simulink model "SEAMOUR_Sim"  (R2023a)
settings: Solver=ode4  StartTime=0.0  StopTime=12  FixedStep=simulation_ts  MaxStep=0.001  MinStep=0.0001  RelTol=1e-3  EnableMultiTasking=on
values from neighbouring files (symbols this model uses):
  Area_y = [0.0031581,0.024875,0.025026,0.021123,0.021123,0.025026,0.024875,0.037486]    [init_file.m]
  Area_z = [0.0031588,0.028932,0.035488,0.030129,0.030129,0.035488,0.028932,0.039984]    [init_file.m]
  Cd_y = [0.5645,0.5232,0.4085,0.3589,0.3589,0.40849,0.5232,0.4642]    [init_file.m]
  Cd_z = [0.5645,0.52,0.5843,0.533,0.533,0.5843,0.52,0.5238]    [init_file.m]
  Coeff = [xudot, yvdot, zwdot]    [init_file.m]
  gravity = 9.81    [init_file.m]
  m = (4*pi*rho*a*b*b)/3    (= 16.3133743522)    [init_file.m]
  offset = 0.002    [init_file.m]
  percent_y = Area_y/t_y    [init_file.m]
  percent_z = Area_z/t_z    [init_file.m]
  xudot = k1*m    [init_file.m]
undefined symbols (not defined in the file or in its folder): center_body, headmain, headmotorshield, headmount, hindconnection, hindcover, kx_lower, kx_upper, kz_lower, kz_upper, lefthindflipper, lefthindmotor, leftmotor1, leftmotor2, leftmotor3, lf_lower, lf_upper, rf_lower, rf_upper, righthindflipper, righthindmotor, rightmotor1, rightmotor2, rightmotor3, tailmotorshield, tailmount, X, Y, Z
libraries: nesl_utility x208, sm_lib x149
(part 1 of 7)
settings Model: Creator=sk3496  LastModifiedBy=andyc
settings SolverCC: InitialStep=0.0001  ExtrapolationOrder=3  AutoInsertRateTranBlk=on  InsertRTBMode=Never (minimum delay)  MinimalZcImpactIntegration=on
settings DataIOCC: LimitDataPoints=on
settings OptimizationCC: LifeSpan=inf
settings DebuggingCC: ReadBeforeWriteMsg=DisableAll  WriteAfterWriteMsg=DisableAll  WriteAfterReadMsg=DisableAll  AlgebraicLoopMsg=none  MultiTaskDSMMsg=none  UnconnectedInputMsg=warning  UnconnectedOutputMsg=warning  UnconnectedLineMsg=warning  AllowSymbolicDim=off  SFUnexpectedBacktrackingDiag=warning  SFNoUnconditionalDefaultTransitionDiag=warning  SFExecutionAtInitializationDiag=none  ArithmeticOperatorsInVariantConditions=warning
settings ModelReferenceCC: UpdateModelReferenceTargets=IfOutOfDate  EnableRefExpFcnMdlSchedulingChecks=on
settings SFSimCC: SFSimEcho=off  SimUseLocalCustomCode=off  CustomCodeUndefinedFunction=UseInterfaceOnly
settings RTWCC: RTWUseLocalCustomCode=off
settings CodeAppCC: StateflowObjectComments=on
settings GRTTargetCC: TargetLangStandard=C89/C90 (ANSI)
settings ConfigComp: CovMetricSettings=dw  CovSaveCumulativeToWorkspaceVar=on  CovSaveSingleToWorkspaceVar=on  CovExternalEMLEnable=off  CovSFcnEnable=off
settings SimscapeCC: SimscapeNominalValues="[{\"value\":\"10\",\"unit\":\"V\"},{\"value\":\"1\",\"unit\":\"A\"},{\"value\":\"10\",\"unit\":\"N*m\"},{\"value\":\"10\",\"unit\":\"bar\"},{\"value\":\"100\",\"unit\":\"kJ/kg\"},{\"value\":\"1\",\"unit\":\"kW\"},{\"value\":\"300\",\"unit\":\"K\"},{\"value\":\"100\",\"unit\":\"cm^3/s\"},{\"value\":\"1\",\"unit\":\"kN\"},{\"value\":\"1\",\"unit\":\"g/cm^3\"},{\"value\":\"1\",\"unit\":\"l\"},{\"value\":\"1\",\"unit\":\"cm^2\"},{\"value\":\"60\",\"unit\":\"Hz\"}]"  SimscapeLogDataHistory=10000
settings ConfigurationSet: Description=SimMechanics 2G

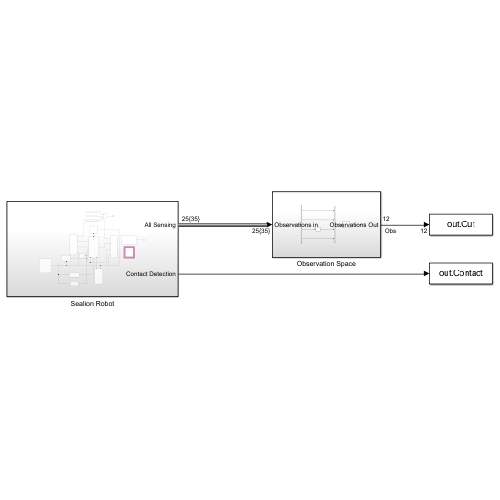
[thumbnail: Simulink's stored preview of the top-level diagram]
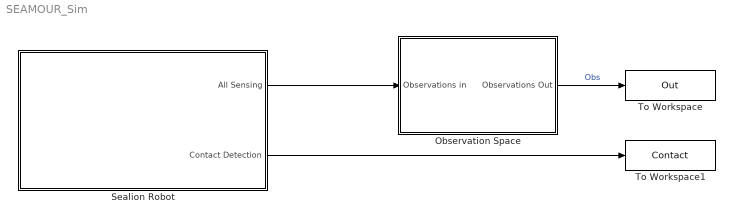
== system SEAMOUR_Sim ==
  Observation Space : Subsystem
  Sealion Robot : Subsystem
  To Workspace : ToWorkspace  VariableName=Out  SaveFormat=Structure  SampleTime=-1
  To Workspace1 : ToWorkspace  VariableName=Contact  SampleTime=-1
      settings: Save2DSignal=2-D array (concatenate along first dimension)
  wires:
  Sealion Robot/1(All Sensing) -> Observation Space/1(Observations in)
  Observation Space/1(Observations Out) -> To Workspace/1  "Obs"
  Sealion Robot/2(Contact Detection) -> To Workspace1/1

== system SEAMOUR_Sim/Observation Space ==
  Observations in : Inport
  Bus Selector : BusSelector  OutputSignals=Body Position/Orientation.Position,Body Position/Orientation.Velocities,Body Position/Orientation.Euler,Body Position/Orientation.AngVel
  Mux : Mux
  Rate Transition : RateTransition
  Reshape1 : Reshape
  Observations Out : Outport
  wires:
  Observations in/1 -> Bus Selector/1
  Bus Selector/3 -> Reshape1/1  "<Euler>"
  Mux/1 -> Rate Transition/1
  Rate Transition/1 -> Observations Out/1
  Bus Selector/1 -> Mux/1  "<Position>"
  Bus Selector/2 -> Mux/2  "<Velocities>"
  Reshape1/1 -> Mux/3
  Bus Selector/4 -> Mux/4  "<AngVel>"

== system SEAMOUR_Sim/Sealion Robot ==
  6 DoF Joint : Subsystem
  All Sesning : Subsystem
  "Allignment Check " : Subsystem
      settings: PortSchema="{\"entries\":[{\"content\":{\"sides\":[{\"content\":{},\"type\":\"ConnectorPlacement.EquallySpacedRectSide\",\"uuid\":\"6b8e2414-6244-4178-ae28-f39780b7a688\"},{\"content\":{\"connectorIds\":[\"RConn1\"],\"side\":\"RIGHT\"},\"type\":\"ConnectorPlacement.EquallySpacedRectSide\",\"uuid\":\"9fd554ac-8ecb-4d79-a032-4bdf23530bdb\"},{\"content\":{\"side\":\"TOP\"},\"type\":\"ConnectorPlacement.EquallySpacedRectSide\",\"uuid\":\"ea6b4beb-e3fc-494d-baa7-bd1cb7ea7a6d\"},{\"content\":{\"connectorIds\":[\"RConn2\"],\"side\":\"BOTTOM\"},\"type\":\"ConnectorPlacement.EquallySpacedRectSide\",\"uuid\":\"7e6024d3-5a2e-46cf-8b0d-4584228e349b\"}]},\"type\":\"ConnectorPlacement.EquallySpacedConnector\",\"uuid\":\"58c9547a-a497-47e7-97e0-14a41819356b\"}],\"packageUris\":[\"http://schema.mathworks.com/mf0/Connector/R2020b\"],\"version\":\"1.0\"}"
  Buoyancy : Subsystem
  Configuration : Subsystem
  Constant : Constant  Value=0
  Distributed Forces : Subsystem
  HEAD : Subsystem
      settings: PortSchema="{\"entries\":[{\"content\":{\"sides\":[{\"content\":{\"connectorIds\":[\"LConn1\"]},\"type\":\"ConnectorPlacement.EquallySpacedRectSide\",\"uuid\":\"8100d47f-b021-448f-a21c-a2dff3a56156\"},{\"content\":{\"side\":\"RIGHT\"},\"type\":\"ConnectorPlacement.EquallySpacedRectSide\",\"uuid\":\"87f545d1-57bd-46af-b957-aab136ed44b5\"},{\"content\":{\"connectorIds\":[\"LConn2\"],\"side\":\"TOP\"},\"type\":\"ConnectorPlacement.EquallySpacedRectSide\",\"uuid\":\"2e5f77fd-6041-45d2-a1f1-1d00d6a46e15\"},{\"content\":{\"side\":\"BOTTOM\"},\"type\":\"ConnectorPlacement.EquallySpacedRectSide\",\"uuid\":\"5c5245d9-55c2-4eb3-8804-cb1ddb21d0c7\"}]},\"type\":\"ConnectorPlacement.EquallySpacedConnector\",\"uuid\":\"e46f37ca-c74f-4ae2-877d-e1d0fe3e0b33\"}],\"packageUris\":[\"http://schema.mathworks.com/mf0/Connector/R2020b\"],\"version\":\"1.0\"}"
      mask Display: image('Icons\Head.PNG')
  LEFT FLIPPER : Subsystem
      settings: PortSchema="{\"entries\":[{\"content\":{\"sides\":[{\"content\":{},\"type\":\"ConnectorPlacement.EquallySpacedRectSide\",\"uuid\":\"08e76363-06a3-4a20-82bd-2cf2d6ca0025\"},{\"content\":{\"side\":\"RIGHT\"},\"type\":\"ConnectorPlacement.EquallySpacedRectSide\",\"uuid\":\"c2e121f7-1b05-4496-8847-526d88e6935b\"},{\"content\":{\"side\":\"TOP\"},\"type\":\"ConnectorPlacement.EquallySpacedRectSide\",\"uuid\":\"ac3d01a4-8d73-45c4-9a34-c3a91121d4c6\"},{\"content\":{\"connectorIds\":[\"RConn1\",\"RConn2\",\"RConn3\",\"RConn4\"],\"side\":\"BOTTOM\"},\"type\":\"ConnectorPlacement.EquallySpacedRectSide\",\"uuid\":\"2a7e8164-9c64-41a5-bf67-24a4b06e045d\"}]},\"type\":\"ConnectorPlacement.EquallySpacedConnector\",\"uuid\":\"d5f6bfd5-69aa-4fea-98cc-f55e388c733b\"}],\"packageUris\":[\"http://schema.mathworks.com/mf0/Connector/R2020b\"],\"version\":\"1.0\"}"
      mask Display: image('Icons\Left_Flipper.PNG')
  PS-Simulink Converter : nesl_utility/PS-Simulink Converter  PhysicalDomain=network_engine_domain  SubClassName=ps_output  LeftPortType=input  RightPortType=output  PseudoPeriodic=off  Frequencies=[]  VectorFormat=inherit  Unit=inherit  AffineConversion=off
  RIGHT FLIPPER : Subsystem
      mask Display: image('Icons\Right_Flipper.PNG')
  Rear : Subsystem
      mask Display: image('Icons\Hind Section.PNG')
  Simulink-PS Converter : nesl_utility/Simulink-PS Converter  PhysicalDomain=network_engine_domain  SubClassName=ps_input  LeftPortType=input  RightPortType=output  PseudoPeriodic=off  Frequencies=[]  NoiseDistribution=none  NoiseParameters=[]  Unit=1  AffineConversion=off  FilteringAndDerivatives=provide  SimscapeFilterOrder=1  InputFilterTimeConstant=0.001  UdotUserProvided=0
  Spatial Contact Force : sm_lib/Forces and Torques/Spatial Contact Force  SenseContactBaseRotation=off  SenseContactBaseTranslation=off  CoefficientOfDynamicFriction=0.3  CoefficientOfStaticFriction=0.5  NormalDamping=1e3  NormalDampingUnits=N/(m/s)  SenseContactSignal=on  NormalStiffness=1e6  NormalStiffnessUnits=N/m  FrictionalCriticalVelocity=1e-3  FrictionalCriticalVelocityUnits=m/s  ZeroCrossDetectContactStartAndEnd=off  SenseContactFollowerRotation=off  SenseContactFollowerTranslation=off  FrictionType=None  SenseFrictionalForceMagnitude=off  SenseNormalForceMagnitude=off  NormalForceType=ProvidedByInput  SenseNormalVelocity=off  SenseSeparationDistance=off  SenseTangentialVelocity=off  NormalTransitionRegionWidth=1e-4  NormalTransitionRegionWidthUnits=m
  Subsystem : Subsystem
      settings: PortSchema="{\"entries\":[{\"content\":{\"sides\":[{\"content\":{\"connectorIds\":[\"LConn1\"]},\"type\":\"ConnectorPlacement.EquallySpacedRectSide\",\"uuid\":\"dcf17234-a2cb-4e8c-ab9b-e151f23c1481\"},{\"content\":{\"connectorIds\":[\"RConn1\",\"RConn2\"],\"side\":\"RIGHT\"},\"type\":\"ConnectorPlacement.EquallySpacedRectSide\",\"uuid\":\"c4f35782-c071-469c-995b-0ee337f7014d\"},{\"content\":{\"connectorIds\":[\"LConn2\"],\"side\":\"TOP\"},\"type\":\"ConnectorPlacement.EquallySpacedRectSide\",\"uuid\":\"5f61ab44-4bc3-42d8-956e-937e7208d291\"},{\"content\":{\"connectorIds\":[\"RConn3\",\"RConn4\",\"RConn5\"],\"side\":\"BOTTOM\"},\"type\":\"ConnectorPlacement.EquallySpacedRectSide\",\"uuid\":\"463c5b41-6d5a-4342-9fda-0edfa9c3fa23\"}]},\"type\":\"ConnectorPlacement.EquallySpacedConnector\",\"uuid\":\"cfa1c9cb-cfd7-41ad-9d03-2a28f55bccb4\"}],\"packageUris\":[\"http://schema.mathworks.com/mf0/Connector/R2020b\"],\"version\":\"1.0\"}"
      mask Display: image('Icons\Center Body.PNG')
  Sum : Sum  Inputs=+++
  Trajectory Inputs : Subsystem
  All Sensing : Outport
  Contact Detection : Outport  Port=2
  wires:
  All Sesning/1(All Sensing) -> All Sensing/1
  Constant/1 -> Simulink-PS Converter/1
  PS-Simulink Converter/1 -> Sum/3
  [Right_Foreflipper_Contact] -> Sum/2
  [Left_Foreflipper_Contact] -> Sum/1
  Sum/1 -> Contact Detection/1
  connections:
  RIGHT FLIPPER/LConn2 -- Subsystem/LConn1
  LEFT FLIPPER/RConn3 -- Subsystem/RConn1
  Buoyancy/LConn1 -- 6 DoF Joint/RConn1 -- "Allignment Check "/RConn1 -- Subsystem/RConn2
  Rear/LConn1 -- Subsystem/RConn3
  HEAD/LConn2 -- Subsystem/LConn2
  Configuration/RConn1 -- HEAD/LConn1 -- RIGHT FLIPPER/LConn4 -- Rear/LConn2 -- LEFT FLIPPER/RConn1 -- "Allignment Check "/RConn2 -- 6 DoF Joint/LConn1 -- Distributed Forces/RConn1
  Distributed Forces/LConn1 -- Subsystem/RConn4
  Subsystem/RConn5 -- LEFT FLIPPER/RConn2 -- RIGHT FLIPPER/LConn3
  Simulink-PS Converter/RConn1 -- Spatial Contact Force/LConn2
  RIGHT FLIPPER/LConn1 -- Spatial Contact Force/RConn1
  PS-Simulink Converter/LConn1 -- Spatial Contact Force/RConn2
  LEFT FLIPPER/RConn4 -- Spatial Contact Force/LConn1

== system SEAMOUR_Sim/Sealion Robot/6 DoF Joint ==
  6-DOF Joint1 : sm_lib/Joints/6-DOF Joint  JointMode=Normal  SenseConstraintForce=off  SenseConstraintForceX=off  SenseConstraintForceY=off  SenseConstraintForceZ=off  SenseConstraintTorque=off  SenseConstraintTorqueX=off  SenseConstraintTorqueY=off  SenseConstraintTorqueZ=off  SenseTotalForce=off  SenseTotalForceX=off  SenseTotalForceY=off  SenseTotalForceZ=off  SenseTotalTorque=off  SenseTotalTorqueX=off  SenseTotalTorqueY=off  SenseTotalTorqueZ=off  CompositeWrenchDir=FollowerOnBase  CompositeWrenchFrame=BaseFrame  PxEquilibriumPosition=0  PxEquilibriumPositionUnits=m  PxSpringStiffness=0  PxSpringStiffnessUnits=N/m  PxDampingCoefficient=0  PxDampingCoefficientUnits=N/(m/s)  PxTorqueActuationMode=NoTorque  PxMotionActuationMode=ComputedMotion  PxSensePosition=on  PxSenseVelocity=on  PxSenseAcceleration=on  PxSenseTorqueForce=off  PxSenseLowerLimitTorqueForce=off  PxSenseUpperLimitTorqueForce=off  PxLowerLimitSpecify=off  PxLowerLimitBound=-1  PxLowerLimitBoundUnits=m  PxLowerLimitStiffness=1e6  PxLowerLimitStiffnessUnits=N/m  PxLowerLimitDamping=1e3  PxLowerLimitDampingUnits=N/(m/s)  PxLowerLimitTransitionRegionWidth=1e-4  PxLowerLimitTransitionRegionWidthUnits=m  PxUpperLimitSpecify=off  PxUpperLimitBound=1  PxUpperLimitBoundUnits=m  PxUpperLimitStiffness=1e6  PxUpperLimitStiffnessUnits=N/m  PxUpperLimitDamping=1e3  PxUpperLimitDampingUnits=N/(m/s)  PxUpperLimitTransitionRegionWidth=1e-4  PxUpperLimitTransitionRegionWidthUnits=m  PxPositionTargetSpecify=off  PxPositionTargetPriority=High  PxPositionTargetValue=0  PxPositionTargetValueUnits=m  PxVelocityTargetSpecify=on  PxVelocityTargetPriority=High  PxVelocityTargetValue=testvel  PxVelocityTargetValueUnits=m/s  PyEquilibriumPosition=0  PyEquilibriumPositionUnits=m  PySpringStiffness=0  PySpringStiffnessUnits=N/m  PyDampingCoefficient=0  PyDampingCoefficientUnits=N/(m/s)  PyTorqueActuationMode=NoTorque  PyMotionActuationMode=ComputedMotion  PySensePosition=on  PySenseVelocity=on  PySenseAcceleration=on  PySenseTorqueForce=off  PySenseLowerLimitTorqueForce=off  PySenseUpperLimitTorqueForce=off  PyLowerLimitSpecify=off  PyLowerLimitBound=-1  PyLowerLimitBoundUnits=m  PyLowerLimitStiffness=1e6  PyLowerLimitStiffnessUnits=N/m  PyLowerLimitDamping=1e3  PyLowerLimitDampingUnits=N/(m/s)  PyLowerLimitTransitionRegionWidth=1e-4  PyLowerLimitTransitionRegionWidthUnits=m  PyUpperLimitSpecify=off  PyUpperLimitBound=1  PyUpperLimitBoundUnits=m  PyUpperLimitStiffness=1e6  PyUpperLimitStiffnessUnits=N/m  PyUpperLimitDamping=1e3  PyUpperLimitDampingUnits=N/(m/s)  PyUpperLimitTransitionRegionWidth=1e-4  PyUpperLimitTransitionRegionWidthUnits=m  PyPositionTargetSpecify=off  PyPositionTargetPriority=High  PyPositionTargetValue=0  PyPositionTargetValueUnits=m  PyVelocityTargetSpecify=off  PyVelocityTargetPriority=High  PyVelocityTargetValue=0  PyVelocityTargetValueUnits=m/s  PzEquilibriumPosition=0  PzEquilibriumPositionUnits=m  PzSpringStiffness=0  PzSpringStiffnessUnits=N/m  PzDampingCoefficient=0  PzDampingCoefficientUnits=N/(m/s)  PzTorqueActuationMode=NoTorque  PzMotionActuationMode=ComputedMotion  PzSensePosition=on  PzSenseVelocity=on  PzSenseAcceleration=on  PzSenseTorqueForce=off  PzSenseLowerLimitTorqueForce=off  PzSenseUpperLimitTorqueForce=off  PzLowerLimitSpecify=off  PzLowerLimitBound=-1  PzLowerLimitBoundUnits=m  PzLowerLimitStiffness=1e6  PzLowerLimitStiffnessUnits=N/m  PzLowerLimitDamping=1e3  PzLowerLimitDampingUnits=N/(m/s)  PzLowerLimitTransitionRegionWidth=1e-4  PzLowerLimitTransitionRegionWidthUnits=m  PzUpperLimitSpecify=off  PzUpperLimitBound=1  PzUpperLimitBoundUnits=m  PzUpperLimitStiffness=1e6  PzUpperLimitStiffnessUnits=N/m  PzUpperLimitDamping=1e3  PzUpperLimitDampingUnits=N/(m/s)  PzUpperLimitTransitionRegionWidth=1e-4  PzUpperLimitTransitionRegionWidthUnits=m  PzPositionTargetSpecify=off  PzPositionTargetPriority=High  PzPositionTargetValue=0  PzPositionTargetValueUnits=m  PzVelocityTargetSpecify=off  PzVelocityTargetPriority=High  PzVelocityTargetValue=0  PzVelocityTargetValueUnits=m/s  SphEqPosRotationMethod=None  SphEqPosRotationAngleUnits=deg  SphEqPosRotationStandardAxis=+Z  SphEqPosRotationAngle=0.0  SphEqPosRotationArbitraryAxis=[0 0 1]  SphEqPosFollAlignAxisA=+X  SphEqPosBaseAlignAxisA=+Y  SphEqPosFollAlignAxisB=+Y  SphEqPosBaseAlignAxisB=+Z  SphEqPosRotationSequenceAxes=FollowerAxes  SphEqPosRotationSequence=XYX  SphEqPosRotationSequenceAngles=[0 0 0]  SphEqPosRotationSequenceAnglesUnits=deg  SphEqPosRotationMatrix=[1 0 0; 0 1 0; 0 0 1]  SphEqPosQuaternion=[1 0 0 0]  SphSpringStiffness=0  SphSpringStiffnessUnits=N*m/deg  SphDampingCoefficient=0  SphDampingCoefficientUnits=N*m/(deg/s)  SphActuateTorqueX=off  SphActuateTorqueY=off  SphActuateTorqueZ=off  SphActuateTorque=off  SphTorqueActuationMode=NoTorque  SphMotionActuationMode=ComputedMotion  SphActuationFrame=BaseFrame  SphSensePosition=on  SphSenseVelocityX=on  SphSenseVelocityY=on  SphSenseVelocityZ=on  SphSenseVelocity=off  SphSenseAccelerationX=off  SphSenseAccelerationY=off  SphSenseAccelerationZ=off  SphSenseAcceleration=off  SphSenseTorqueX=off  SphSenseTorqueY=off  SphSenseTorqueZ=off  SphSenseTorqueForce=off  SphSenseLowerLimitTorqueMag=off  SphSenseUpperLimitTorqueMag=off  SphSensingFrame=BaseFrame  SphLowerLimitSpecify=off  SphLowerLimitBound=15  SphLowerLimitBoundUnits=deg  SphLowerLimitStiffness=1e4  SphLowerLimitStiffnessUnits=N*m/deg  SphLowerLimitDamping=10  SphLowerLimitDampingUnits=N*m/(deg/s)  SphLowerLimitTransitionRegionWidth=0.1  SphLowerLimitTransitionRegionWidthUnits=deg  SphUpperLimitSpecify=off  SphUpperLimitBound=45  SphUpperLimitBoundUnits=deg  SphUpperLimitStiffness=1e4  SphUpperLimitStiffnessUnits=N*m/deg  SphUpperLimitDamping=10  SphUpperLimitDampingUnits=N*m/(deg/s)  SphUpperLimitTransitionRegionWidth=0.1  SphUpperLimitTransitionRegionWidthUnits=deg  SphPositionTargetRotationMethod=None  SphPositionTargetRotationAngleUnits=deg  SphPositionTargetRotationStandardAxis=+Z  SphPositionTargetRotationAngle=0.0  SphPositionTargetRotationArbitraryAxis=[0 0 1]  SphPositionTargetFollAlignAxisA=+X  SphPositionTargetBaseAlignAxisA=+Y  SphPositionTargetFollAlignAxisB=+Y  SphPositionTargetBaseAlignAxisB=+Z  SphPositionTargetRotationSequenceAxes=FollowerAxes  SphPositionTargetRotationSequence=XYX  SphPositionTargetRotationSequenceAngles=[0 0 0]  SphPositionTargetRotationSequenceAnglesUnits=deg  SphPositionTargetRotationMatrix=[1 0 0; 0 1 0; 0 0 1]  SphPositionTargetQuaternion=[1 0 0 0]  SphPositionTargetSpecify=off  SphPositionTargetPriority=High  SphVelocityTargetValue=[0 0 0]  SphVelocityTargetValueUnits=deg/s  SphVelocityTargetSpecify=off  SphVelocityTargetPriority=High  SphVelocityTargetInFollowerFrame=on
  Bus Creator : BusCreator  Inputs=5
  MATLAB Function : MATLAB Function  TreatAsAtomicUnit=on
  Mux{,1..3} (4 alike) : Mux  Inputs=3
  PS-Simulink Converter{1..13} (13 alike) : nesl_utility/PS-Simulink Converter  PhysicalDomain=network_engine_domain  SubClassName=ps_output  LeftPortType=input  RightPortType=output  PseudoPeriodic=off  Frequencies=[]  VectorFormat=1-D array  Unit=1  AffineConversion=off
  World Frame : PMIOPort  Side=Left
  To CoM : PMIOPort  Port=2  Side=Right
  tag scope: Body_Kinematics=global
  wires:
  PS-Simulink Converter13/1 -> Mux3/1  "wx"
  PS-Simulink Converter1/1 -> Mux1/1  "vx"
  Mux3/1 -> Bus Creator/5  "AngVel"
  PS-Simulink Converter8/1 -> MATLAB Function/1(u)  "Orientation"
  PS-Simulink Converter11/1 -> Mux2/3  "az"
  Mux2/1 -> Bus Creator/3  "Accelerations"
  PS-Simulink Converter3/1 -> Mux/2  "px"
  PS-Simulink Converter12/1 -> Mux3/2  "wy"
  PS-Simulink Converter9/1 -> Mux2/1  "ax"
  PS-Simulink Converter10/1 -> Mux/1  "px"
  PS-Simulink Converter2/1 -> Mux1/2  "vy"
  PS-Simulink Converter6/1 -> Mux/3  "pz"
  Mux/1 -> Bus Creator/1  "Position"
  PS-Simulink Converter4/1 -> Mux2/2  "ay"
  PS-Simulink Converter7/1 -> Mux3/3  "wz"
  PS-Simulink Converter5/1 -> Mux1/3  "vz"
  Mux1/1 -> Bus Creator/2  "Velocities"
  Bus Creator/1 -> [Body_Kinematics]
  MATLAB Function/1(y) -> Bus Creator/4  "Euler"
  connections:
  6-DOF Joint1/RConn12 -- PS-Simulink Converter13/LConn1
  To CoM/RConn1 -- 6-DOF Joint1/RConn1
  6-DOF Joint1/RConn6 -- PS-Simulink Converter2/LConn1
  6-DOF Joint1/RConn14 -- PS-Simulink Converter7/LConn1
  6-DOF Joint1/RConn4 -- PS-Simulink Converter9/LConn1
  6-DOF Joint1/RConn8 -- PS-Simulink Converter6/LConn1
  6-DOF Joint1/RConn3 -- PS-Simulink Converter1/LConn1
  6-DOF Joint1/RConn11 -- PS-Simulink Converter8/LConn1
  6-DOF Joint1/RConn13 -- PS-Simulink Converter12/LConn1
  6-DOF Joint1/RConn7 -- PS-Simulink Converter4/LConn1
  6-DOF Joint1/RConn2 -- PS-Simulink Converter10/LConn1
  6-DOF Joint1/RConn9 -- PS-Simulink Converter5/LConn1
  6-DOF Joint1/RConn5 -- PS-Simulink Converter3/LConn1
  6-DOF Joint1/RConn10 -- PS-Simulink Converter11/LConn1
  World Frame/RConn1 -- 6-DOF Joint1/LConn1

== system SEAMOUR_Sim/Sealion Robot/All Sesning ==
  Bus Creator : BusCreator  Inputs=3
  Bus Creator1 : BusCreator  Inputs=6
  Bus Creator2 : BusCreator  Inputs=14
  All Sensing : Outport
  wires:
  [left_roll_power] -> Bus Creator1/3  "Left Roll Power"
  [left_yaw_power] -> Bus Creator1/2  "Left Yaw Power"
  [right_pitch_power] -> Bus Creator1/4  "Right Pitch Power"
  Bus Creator1/1 -> Bus Creator/2  "Flipper Power"
  [right_roll_power] -> Bus Creator1/6  "Right Roll Power"
  [left_pitch_power] -> Bus Creator1/1  "Left Pitch Power"
  [right_yaw_power] -> Bus Creator1/5  "Right Yaw Power"
  [Body_Kinematics] -> Bus Creator/1  "Body Position/Orientation"
  Bus Creator/1 -> All Sensing/1
  [head_pitch_position] -> Bus Creator2/1  "head pitch"
  [head_yaw_position] -> Bus Creator2/2  "head yaw"
  [left_fore_pitch_position] -> Bus Creator2/3  "left fore pitch"
  [left_fore_yaw_position] -> Bus Creator2/4  "left fore yaw"
  [left_fore_roll_position] -> Bus Creator2/5  "left fore roll"
  [right_fore_pitch_position] -> Bus Creator2/6  "right fore pitch"
  [right_fore_yaw_position] -> Bus Creator2/7  "right fore yaw"
  [right_fore_roll_position] -> Bus Creator2/8  "right fore roll"
  [hind_pitch_position] -> Bus Creator2/9  "hind pitch"
  [hind_yaw_position] -> Bus Creator2/10  "hind yaw"
  [left_hind_yaw_position] -> Bus Creator2/11  "left hind yaw"
  [left_hind_roll_position] -> Bus Creator2/12  "left hind roll"
  [right_hind_yaw_position] -> Bus Creator2/13  "right hind yaw"
  [right_hind_roll_position] -> Bus Creator2/14  "right hind roll"
  Bus Creator2/1 -> Bus Creator/3  "Actuator Positions"

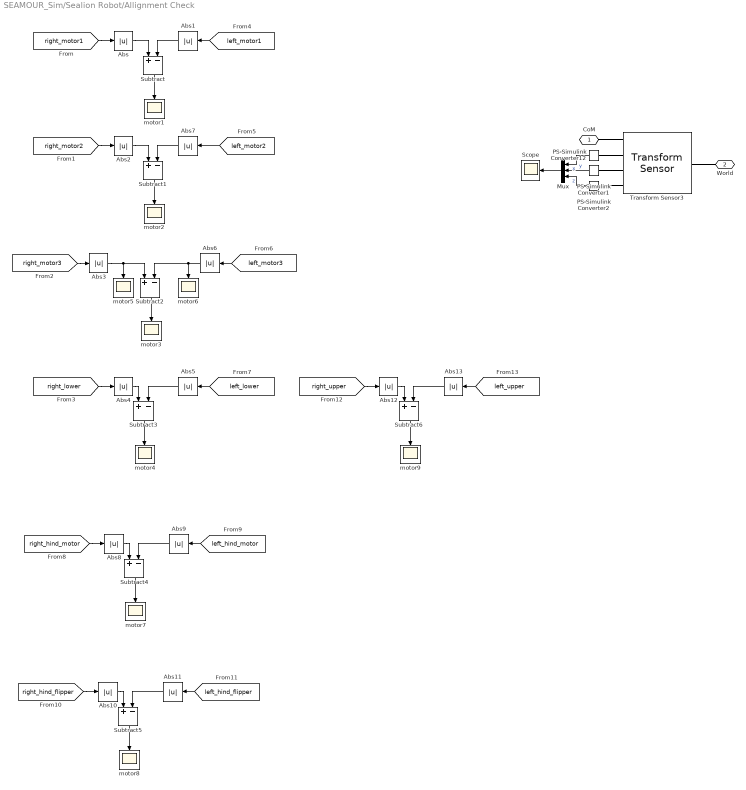
== system SEAMOUR_Sim/Sealion Robot/Allignment Check  ==
  Abs{,1..13} (14 alike) : Abs  SaturateOnIntegerOverflow=off
  Mux : Mux  Inputs=3
  PS-Simulink Converter1 : nesl_utility/PS-Simulink Converter  PhysicalDomain=network_engine_domain  SubClassName=ps_output  LeftPortType=input  RightPortType=output  PseudoPeriodic=off  Frequencies=[]  VectorFormat=1-D array  Unit=1  AffineConversion=off
  PS-Simulink Converter12 : nesl_utility/PS-Simulink Converter  PhysicalDomain=network_engine_domain  SubClassName=ps_output  LeftPortType=input  RightPortType=output  PseudoPeriodic=off  Frequencies=[]  VectorFormat=1-D array  Unit=1  AffineConversion=off
  PS-Simulink Converter2 : nesl_utility/PS-Simulink Converter  PhysicalDomain=network_engine_domain  SubClassName=ps_output  LeftPortType=input  RightPortType=output  PseudoPeriodic=off  Frequencies=[]  VectorFormat=1-D array  Unit=1  AffineConversion=off
  Scope : Scope
  Subtract{,1..6} (7 alike) : Sum  Inputs=+-
  Transform Sensor3 : sm_lib/Frames and Transforms/Transform Sensor  MeasurementFrame=NonRotatingFollower  RotationSequence=XYX  SenseAngle=off  SenseAxis=off  SenseQ=off  SenseR=off  SenseRotationSequence=off  SenseOmegaX=off  SenseOmegaY=off  SenseOmegaZ=off  SenseQDot=off  SenseRDot=off  SenseRotationSequenceDot=off  SenseAlphaX=off  SenseAlphaY=off  SenseAlphaZ=off  SenseQDDot=off  SenseRDDot=off  SenseX=on  SenseY=on  SenseZ=on  SenseRad=off  SenseAzim=off  SenseDist=off  SenseInc=off  SenseXDot=off  SenseYDot=off  SenseZDot=off  SenseRadDot=off  SenseAzimDot=off  SenseDistDot=off  SenseIncDot=off  SenseXDDot=off  SenseYDDot=off  SenseZDDot=off  SenseRadDDot=off  SenseAzimDDot=off  SenseDistDDot=off  SenseIncDDot=off
  motor{1..9} (9 alike) : Scope
  CoM : PMIOPort  Side=Right
  World : PMIOPort  Port=2  Side=Right
  wires:
  Subtract/1 -> motor1/1
  [right_motor1] -> Abs/1
  [left_motor1] -> Abs1/1
  Subtract1/1 -> motor2/1
  [left_motor2] -> Abs7/1
  [right_motor2] -> Abs2/1
  [right_motor3] -> Abs3/1
  Subtract2/1 -> motor3/1
  [right_lower] -> Abs4/1
  Subtract3/1 -> motor4/1
  [left_lower] -> Abs5/1
  Abs/1 -> Subtract/1
  Abs1/1 -> Subtract/2
  Abs2/1 -> Subtract1/1
  Abs3/1 -> motor5/1, Subtract2/1
  Abs4/1 -> Subtract3/1
  Abs5/1 -> Subtract3/2
  Abs6/1 -> motor6/1, Subtract2/2
  Abs7/1 -> Subtract1/2
  PS-Simulink Converter1/1 -> Mux/2  "y"
  PS-Simulink Converter12/1 -> Mux/1  "x"
  PS-Simulink Converter2/1 -> Mux/3  "z"
  Mux/1 -> Scope/1
  [left_motor3] -> Abs6/1
  Abs8/1 -> Subtract4/1
  Subtract4/1 -> motor7/1
  Abs9/1 -> Subtract4/2
  [left_hind_motor] -> Abs9/1
  [right_hind_motor] -> Abs8/1
  [left_hind_flipper] -> Abs11/1
  [right_hind_flipper] -> Abs10/1
  Abs11/1 -> Subtract5/2
  Subtract5/1 -> motor8/1
  Abs10/1 -> Subtract5/1
  [right_upper] -> Abs12/1
  [left_upper] -> Abs13/1
  Abs13/1 -> Subtract6/2
  Subtract6/1 -> motor9/1
  Abs12/1 -> Subtract6/1
  connections:
  PS-Simulink Converter2/LConn1 -- Transform Sensor3/RConn4
  PS-Simulink Converter12/LConn1 -- Transform Sensor3/RConn2
  PS-Simulink Converter1/LConn1 -- Transform Sensor3/RConn3
  World/RConn1 -- Transform Sensor3/LConn1
  CoM/RConn1 -- Transform Sensor3/RConn1

== system SEAMOUR_Sim/Sealion Robot/Buoyancy ==
  Buoyancy (N) : Constant  Value=center_body.mass*gravity
  Fz on the CoB : sm_lib/Forces and Torques/External Force and Torque  ForceResolutionFrame=World  EnableForceX=off  EnableForceY=on  EnableForceZ=off  EnableForce=off  TorqueResolutionFrame=World  EnableTorqueX=off  EnableTorqueY=off  EnableTorqueZ=off  EnableTorque=off
  Gain : Gain
  Rigid Transform : sm_lib/Frames and Transforms/Rigid Transform  TranslationMethod=Cartesian  TranslationStandardOffset=0  TranslationStandardOffsetUnits=m  TranslationStandardAxis=+Z  TranslationCartesianOffset=[0 0 offset]  TranslationCartesianOffsetUnits=m  TranslationROffset=0  TranslationROffsetUnits=m  TranslationZOffset=0  TranslationZOffsetUnits=m  TranslationThetaOffset=0  TranslationThetaOffsetUnits=deg  RotationMethod=None  RotationAngleUnits=deg  RotationStandardAxis=+Z  RotationAngle=0.0  RotationArbitraryAxis=[0 0 1]  FollAlignAxisA=+X  BaseAlignAxisA=+Y  FollAlignAxisB=+Y  BaseAlignAxisB=+Z  RotationSequenceAxes=FollowerAxes  RotationSequence=XYX  RotationSequenceAngles=[0 0 0]  RotationSequenceAnglesUnits=deg  RotationMatrix=[1 0 0; 0 1 0; 0 0 1]  Quaternion=[1 0 0 0]
  SPS3 : nesl_utility/Simulink-PS Converter  PhysicalDomain=network_engine_domain  SubClassName=ps_input  LeftPortType=input  RightPortType=output  PseudoPeriodic=off  Frequencies=[]  NoiseDistribution=none  NoiseParameters=[]  Unit=N  AffineConversion=off  FilteringAndDerivatives=provide  SimscapeFilterOrder=1  InputFilterTimeConstant=0.001  UdotUserProvided=0
  To CoM : PMIOPort  Side=Left
  wires:
  Buoyancy (N)/1 -> Gain/1
  Gain/1 -> SPS3/1
  connections:
  Rigid Transform/LConn1 -- To CoM/RConn1
  Fz on the CoB/LConn1 -- SPS3/RConn1
  Rigid Transform/RConn1 -- Fz on the CoB/RConn1

== system SEAMOUR_Sim/Sealion Robot/Configuration ==
  Mechanism Configuration : sm_lib/Utilities/Mechanism Configuration  UniformGravity=Constant  GravityVector=[0 -9.81 0]  GravityVectorUnits=m/s^2  LinearizationDelta=0.001  JointModeTransitionNonlinearIterations=2
  Rigid Transform15 : sm_lib/Frames and Transforms/Rigid Transform  TranslationMethod=Cartesian  TranslationStandardOffset=0  TranslationStandardOffsetUnits=mm  TranslationStandardAxis=+Z  TranslationCartesianOffset=[0 0 0]  TranslationCartesianOffsetUnits=mm  TranslationROffset=0  TranslationROffsetUnits=m  TranslationZOffset=0  TranslationZOffsetUnits=m  TranslationThetaOffset=0  TranslationThetaOffsetUnits=deg  RotationMethod=StandardAxis  RotationAngleUnits=deg  RotationStandardAxis=-Y  RotationAngle=90  RotationArbitraryAxis=[0 0 1]  FollAlignAxisA=+X  BaseAlignAxisA=+Y  FollAlignAxisB=+Y  BaseAlignAxisB=+Z  RotationSequenceAxes=FollowerAxes  RotationSequence=XYX  RotationSequenceAngles=[0 0 0]  RotationSequenceAnglesUnits=deg  RotationMatrix=[1 0 0; 0 1 0; 0 0 1]  Quaternion=[1 0 0 0]
  Rigid Transform16 : sm_lib/Frames and Transforms/Rigid Transform  TranslationMethod=Cartesian  TranslationStandardOffset=0  TranslationStandardOffsetUnits=mm  TranslationStandardAxis=+Z  TranslationCartesianOffset=[0 0 0]  TranslationCartesianOffsetUnits=mm  TranslationROffset=0  TranslationROffsetUnits=m  TranslationZOffset=0  TranslationZOffsetUnits=m  TranslationThetaOffset=0  TranslationThetaOffsetUnits=deg  RotationMethod=StandardAxis  RotationAngleUnits=deg  RotationStandardAxis=-X  RotationAngle=90  RotationArbitraryAxis=[0 0 1]  FollAlignAxisA=+X  BaseAlignAxisA=+Y  FollAlignAxisB=+Y  BaseAlignAxisB=+Z  RotationSequenceAxes=FollowerAxes  RotationSequence=XYX  RotationSequenceAngles=[0 0 0]  RotationSequenceAnglesUnits=deg  RotationMatrix=[1 0 0; 0 1 0; 0 0 1]  Quaternion=[1 0 0 0]
  Solver Configuration : nesl_utility/Solver Configuration  PhysicalDomain=network_engine_domain  SubClassName=solver  LeftPortType=input  RightPortType=generic  Tones=[]  Harmonics=[]  SimulateNoise=off  Profile=off  UseLocalSampling=off  EnableSwitchedLinearOptims=on  FrequencyDomain=off  UseCCode=off  RelTol=0.001  AbsTol=1e-06  MinStep=1e-09  ToWorkspace=off  RevertToSquareIcSolve=off  NumHomotopyIterations=100  PhasorMode=off  PhasorModeNumHarmonics=1  ConsistencySolver=NEWTON_XTOL_AFTER_FTOL  IndexReductionMethod=DerivativeReplacement  DoDC=off  ResidualTolerance=1e-9  ConsistencyTolSource=GLOBAL  ConsistencyAbsTol=0.001  ConsistencyRelTol=0.001  ConsistencyTolFactor=0.001  UseLocalSolver=off  LocalSolverChoice=NE_BACKWARD_EULER_ADVANCER  ResolveIndetEquations=on  FunctionEvalNumThread=1  LocalSolverSampleTime=.001  DoFixedCost=off  MaxNonlinIter=3  MaxModeIter=2  ComputeImpulses=off  ImpulseIterations=2  LinearAlgebra=auto  LinearAlgebraNumThread=0  EquationFormulation=NE_TIME_EF  DelaysMemoryBudget=1024  AutomaticFiltering=on  FilteringTimeConstant=0.001  PartitionStorageMethod=AS_NEEDED  PartitionMemoryBudget=1024  PartitionMethod=FAST
  World Frame : sm_lib/Frames and Transforms/World Frame
  Configuration Block : PMIOPort  Side=Right
  connections:
  Mechanism Configuration/RConn1 -- Solver Configuration/RConn1 -- Rigid Transform15/LConn1 -- World Frame/RConn1
  Rigid Transform16/RConn1 -- Configuration Block/RConn1
  Rigid Transform15/RConn1 -- Rigid Transform16/LConn1

== system SEAMOUR_Sim/Sealion Robot/Distributed Forces ==
  Added Mass in X : Subsystem
  Distbuted Load In y and z directions : Subsystem
  Drag force in x direction : Subsystem
  To Ref : PMIOPort  Side=Left
  World Frame : PMIOPort  Port=2  Side=Right
  connections:
  Added Mass in X/LConn1 -- Drag force in x direction/LConn1 -- World Frame/RConn1 -- Distbuted Load In y and z directions/LConn1
  Distbuted Load In y and z directions/RConn1 -- Added Mass in X/RConn2 -- Added Mass in X/RConn1 -- To Ref/RConn1 -- Drag force in x direction/RConn1 -- Drag force in x direction/RConn2

== system SEAMOUR_Sim/Sealion Robot/HEAD ==
  Head : Subsystem
  Mux : Mux  Inputs=3
  PS-Simulink Converter : nesl_utility/PS-Simulink Converter  PhysicalDomain=network_engine_domain  SubClassName=ps_output  LeftPortType=input  RightPortType=output  PseudoPeriodic=off  Frequencies=[]  VectorFormat=inherit  Unit=inherit  AffineConversion=off
  PS-Simulink Converter1 : nesl_utility/PS-Simulink Converter  PhysicalDomain=network_engine_domain  SubClassName=ps_output  LeftPortType=input  RightPortType=output  PseudoPeriodic=off  Frequencies=[]  VectorFormat=inherit  Unit=inherit  AffineConversion=off
  PS-Simulink Converter2 : nesl_utility/PS-Simulink Converter  PhysicalDomain=network_engine_domain  SubClassName=ps_output  LeftPortType=input  RightPortType=output  PseudoPeriodic=off  Frequencies=[]  VectorFormat=inherit  Unit=inherit  AffineConversion=off
  Rigid Transform : sm_lib/Frames and Transforms/Rigid Transform  TranslationMethod=Cartesian  TranslationStandardOffset=0  TranslationStandardOffsetUnits=m  TranslationStandardAxis=+Z  TranslationCartesianOffset=[0 0.000519615242261 -0.000000000000355]  TranslationCartesianOffsetUnits=m  TranslationROffset=0  TranslationROffsetUnits=m  TranslationZOffset=0  TranslationZOffsetUnits=m  TranslationThetaOffset=0  TranslationThetaOffsetUnits=deg  RotationMethod=StandardAxis  RotationAngleUnits=deg  RotationStandardAxis=+X  RotationAngle=180  RotationArbitraryAxis=[0 0 1]  FollAlignAxisA=+X  BaseAlignAxisA=+Y  FollAlignAxisB=+Y  BaseAlignAxisB=+Z  RotationSequenceAxes=FollowerAxes  RotationSequence=XYX  RotationSequenceAngles=[0 0 0]  RotationSequenceAnglesUnits=deg  RotationMatrix=[1 0 0; 0 1 0; 0 0 1]  Quaternion=[1 0 0 0]
  To Workspace : ToWorkspace  VariableName=head_offset  SampleTime=-1
      settings: Save2DSignal=2-D array (concatenate along first dimension)
  Transform Sensor : sm_lib/Frames and Transforms/Transform Sensor  MeasurementFrame=World  RotationSequence=XYX  SenseAngle=off  SenseAxis=off  SenseQ=off  SenseR=off  SenseRotationSequence=off  SenseOmegaX=off  SenseOmegaY=off  SenseOmegaZ=off  SenseQDot=off  SenseRDot=off  SenseRotationSequenceDot=off  SenseAlphaX=off  SenseAlphaY=off  SenseAlphaZ=off  SenseQDDot=off  SenseRDDot=off  SenseX=on  SenseY=on  SenseZ=on  SenseRad=off  SenseAzim=off  SenseDist=off  SenseInc=off  SenseXDot=off  SenseYDot=off  SenseZDot=off  SenseRadDot=off  SenseAzimDot=off  SenseDistDot=off  SenseIncDot=off  SenseXDDot=off  SenseYDDot=off  SenseZDDot=off  SenseRadDDot=off  SenseAzimDDot=off  SenseDistDDot=off  SenseIncDDot=off
  to world frame : PMIOPort  Side=Left
  To Center : PMIOPort  Port=2  Side=Left
  wires:
  PS-Simulink Converter/1 -> Mux/1
  PS-Simulink Converter1/1 -> Mux/2
  PS-Simulink Converter2/1 -> Mux/3
  Mux/1 -> To Workspace/1
  connections:
  Transform Sensor/LConn1 -- to world frame/RConn1 -- Head/LConn3
  PS-Simulink Converter/LConn1 -- Transform Sensor/RConn2
  PS-Simulink Converter1/LConn1 -- Transform Sensor/RConn3
  PS-Simulink Converter2/LConn1 -- Transform Sensor/RConn4
  Rigid Transform/LConn1 -- To Center/RConn1
  Head/LConn1 -- Rigid Transform/RConn1
  Transform Sensor/RConn1 -- Head/LConn2

== system SEAMOUR_Sim/Sealion Robot/LEFT FLIPPER ==
  Left Motors : Subsystem
  Subsystem : Subsystem
      settings: PortSchema="{\"entries\":[{\"content\":{\"sides\":[{\"content\":{\"connectorIds\":[\"LConn1\",\"LConn2\"]},\"type\":\"ConnectorPlacement.EquallySpacedRectSide\",\"uuid\":\"934c01b4-1c58-4ffc-b615-75f709d3e62f\"},{\"content\":{\"side\":\"RIGHT\"},\"type\":\"ConnectorPlacement.EquallySpacedRectSide\",\"uuid\":\"537d3515-7ad3-498d-b808-21221918efc9\"},{\"content\":{\"side\":\"TOP\"},\"type\":\"ConnectorPlacement.EquallySpacedRectSide\",\"uuid\":\"93cf9426-a9f3-4142-8d37-60e304b7cc37\"},{\"content\":{\"connectorIds\":[\"RConn1\",\"RConn2\"],\"side\":\"BOTTOM\"},\"type\":\"ConnectorPlacement.EquallySpacedRectSide\",\"uuid\":\"2918a618-4bdd-4454-bf07-eec1ba9ff485\"}]},\"type\":\"ConnectorPlacement.EquallySpacedConnector\",\"uuid\":\"e2472ef9-d08b-4187-9a10-641a47d7d4fd\"}],\"packageUris\":[\"http://schema.mathworks.com/mf0/Connector/R2020b\"],\"version\":\"1.0\"}"
  To World Frame : PMIOPort  Side=Right
  Center Hull Boundary : PMIOPort  Port=2  Side=Right
  To Center : PMIOPort  Port=3  Side=Right
  Left Flipper Boundary : PMIOPort  Port=4  Side=Right
  connections:
  Subsystem/LConn2 -- Left Motors/RConn2 -- To World Frame/RConn1
  Left Motors/RConn1 -- Subsystem/LConn1
  To Center/RConn1 -- Left Motors/LConn1
  Center Hull Boundary/RConn1 -- Subsystem/RConn1
  Left Flipper Boundary/RConn1 -- Subsystem/RConn2

== system SEAMOUR_Sim/Sealion Robot/RIGHT FLIPPER ==
  RIght Motors : Subsystem
      settings: PortSchema="{\"entries\":[{\"content\":{\"sides\":[{\"content\":{\"connectorIds\":[\"LConn1\"]},\"type\":\"ConnectorPlacement.EquallySpacedRectSide\",\"uuid\":\"42f6983b-2dd3-45f1-8f7d-6b75e960b6e1\"},{\"content\":{\"connectorIds\":[\"RConn1\"],\"side\":\"RIGHT\"},\"type\":\"ConnectorPlacement.EquallySpacedRectSide\",\"uuid\":\"3116529c-92c7-4068-81e0-a5193d3addeb\"},{\"content\":{\"side\":\"TOP\"},\"type\":\"ConnectorPlacement.EquallySpacedRectSide\",\"uuid\":\"0797a7b0-8c20-4676-bd42-ddfdf242801d\"},{\"content\":{\"connectorIds\":[\"RConn2\"],\"side\":\"BOTTOM\"},\"type\":\"ConnectorPlacement.EquallySpacedRectSide\",\"uuid\":\"2c0a2851-55bd-4e39-b073-18263d23b146\"}]},\"type\":\"ConnectorPlacement.EquallySpacedConnector\",\"uuid\":\"e6cb51ff-eaef-44c5-ada5-ebb2b25d852e\"}],\"packageUris\":[\"http://schema.mathworks.com/mf0/Connector/R2020b\"],\"version\":\"1.0\"}"
  Subsystem1 : Subsystem
  Right Flipper Boundary : PMIOPort  Side=Left
  To Center : PMIOPort  Port=2  Side=Left
  Center Hull Boundary : PMIOPort  Port=3  Side=Left
  To World Frame : PMIOPort  Port=4  Side=Left
  connections:
  RIght Motors/RConn1 -- Subsystem1/LConn1
  To Center/RConn1 -- RIght Motors/LConn1
  To World Frame/RConn1 -- RIght Motors/RConn2 -- Subsystem1/LConn2
  Center Hull Boundary/RConn1 -- Subsystem1/RConn1
  Subsystem1/RConn2 -- Right Flipper Boundary/RConn1

== system SEAMOUR_Sim/Sealion Robot/Rear ==
  Buoyancy (N) : Constant  Value=hindconnection.mass*gravity
  Fz on the CoB : sm_lib/Forces and Torques/External Force and Torque  ForceResolutionFrame=World  EnableForceX=off  EnableForceY=on  EnableForceZ=off  EnableForce=off  TorqueResolutionFrame=World  EnableTorqueX=off  EnableTorqueY=off  EnableTorqueZ=off  EnableTorque=off
  Hind Flipper Connection : sm_lib/Body Elements/File Solid  ExtGeomFileName=Simscape_Parts_StepFiles/hind_section_motor2.stp  UnitType=FromFile  ExtGeomFileUnits=mm  StepReaderType=HEX  ExportConvexHullGeometry=off  InertiaType=Custom  Mass=hindconnection.mass  MassUnits=kg  CenterOfMass=hindconnection.com  CenterOfMassUnits=m  MomentsOfInertia=hindconnection.inertia  MomentsOfInertiaUnits=kg*m^2  ProductsOfInertia=hindconnection.prodinertia  ProductsOfInertiaUnits=kg*m^2  BasedOnType=DensityFromFile  Density=2.7  DensityUnits=kg/m^3  DoExposeReferenceFrame=off  SerializedFrames=<Frames><Frame><Id>Frame1</Id><Value><Name>to center</Name><Origin><Source>GeometricFeature</Source><FeatureName>circular curve 668</FeatureName></Origin><PrimaryAxis><DefinedDirection>+X</DefinedDirection><Source>ReferenceFrame</Source><SourceDirection>+Z</SourceDirection><FeatureName></FeatureName></PrimaryAxis><SecondaryAxis><DefinedDirection>+Z</DefinedDirection><Source>GeometricFeature</Source><SourceDirection>+X</SourceDirection><FeatureName>planar surface 886</FeatureName></SecondaryAxis></Value></Frame><Frame><Id>Frame2</Id><Value><Name>flipper left</Name><Origin><Source>GeometricFeature</Source><FeatureName>circular curve 4</FeatureName></Origin><PrimaryAxis><DefinedDirection>+X</DefinedDirection><Source>GeometricFeature</Source><SourceDirection>+Z</SourceDirection><FeatureName>segment 1441</FeatureName></PrimaryAxis><SecondaryAxis><DefinedDirection>+Y</DefinedDirection><Source>GeometricFeature</Source><SourceDirection>+X</SourceDirection><FeatureName>segment 1528</FeatureName></SecondaryAxis></Value></Frame><Frame><Id>Frame3</Id><Value><Name>flipper right</Name><Origin><Source>GeometricFeature</Source><FeatureName>circular curve 8</FeatureName></Origin><PrimaryAxis><DefinedDirection>+Y</DefinedDirection><Source>ReferenceFrame</Source><SourceDirection>+X</SourceDirection><FeatureName></FeatureName></PrimaryAxis><SecondaryAxis><DefinedDirection>+Z</DefinedDirection><Source>ReferenceFrame</Source><SourceDirection>+Y</SourceDirection><FeatureName></FeatureName></SecondaryAxis></Value></Frame><Frame><Id>Frame4</Id><Value><Name>Hind Cover</Name><Origin><Source>GeometricFeature</Source><FeatureName>circular curve 906</FeatureName></Origin><PrimaryAxis><DefinedDirection>+X</DefinedDirection><Source>ReferenceFrame</Source><SourceDirection>+Z</SourceDirection><FeatureName></FeatureName></PrimaryAxis><SecondaryAxis><DefinedDirection>+Y</DefinedDirection><Source>ReferenceFrame</Source><SourceDirection>+X</SourceDirection><FeatureName></FeatureName></SecondaryAxis></Value></Frame><Frame><Id>Frame5</Id><Value><Name>CoM</Name><Origin><Source>CenterOfMassFrame</Source><FeatureName></FeatureName></Origin><PrimaryAxis><DefinedDirection>+Y</DefinedDirection><Source>ReferenceFrame</Source><SourceDirection>-Z</SourceDirection><FeatureName></FeatureName></PrimaryAxis><SecondaryAxis><DefinedDirection>+X</DefinedDirection><Source>ReferenceFrame</Source><SourceDirection>+X</SourceDirection><FeatureName></FeatureName></SecondaryAxis></Value></Frame><Frame><Id>Frame6</Id><Value><Name>Allign_Center</Name><Origin><Source>GeometricFeature</Source><FeatureName>circular curve 923</FeatureName></Origin><PrimaryAxis><DefinedDirection>+Z</DefinedDirection><Source>ReferenceFrame</Source><SourceDirection>+Z</SourceDirection><FeatureName></FeatureName></PrimaryAxis><SecondaryAxis><DefinedDirection>+X</DefinedDirection><Source>ReferenceFrame</Source><SourceDirection>+X</SourceDirection><FeatureName></FeatureName></SecondaryAxis></Value></Frame><Frame><Id>Frame7</Id><Value><Name>CoB</Name><Origin><Source>CenterOfMassFrame</Source><FeatureName></FeatureName></Origin><PrimaryAxis><DefinedDirection>+Y</DefinedDirection><Source>ReferenceFrame</Source><SourceDirection>-Z</SourceDirection><FeatureName></FeatureName></PrimaryAxis><SecondaryAxis><DefinedDirection>+X</DefinedDirection><Source>ReferenceFrame</Source><SourceDirection>+X</SourceDirection><FeatureName></FeatureName></SecondaryAxis></Value></Frame></Frames>  GraphicType=FromGeometry  MarkerShape=Sphere  MarkerSize=10  GraphicVisPropType=SimpleVisualProperties  GraphicDiffuseColor=[0.2 0.4 1.0]  GraphicSpecularColor=[0.5 0.5 0.5 1.0]  GraphicAmbientColor=[0.15 0.15 0.15 1.0]  GraphicEmissiveColor=[0.0 0.0 0.0 1.0]  GraphicShininess=75  GraphicOpacity=1.0
  Hind Section Actuators : Subsystem
  Left Hind Flipper : Subsystem
      settings: PortSchema="{\"entries\":[{\"content\":{\"sides\":[{\"content\":{\"connectorIds\":[\"LConn1\"]},\"type\":\"ConnectorPlacement.EquallySpacedRectSide\",\"uuid\":\"81868130-85f8-4e49-a1b3-febf46c0aefa\"},{\"content\":{\"side\":\"RIGHT\"},\"type\":\"ConnectorPlacement.EquallySpacedRectSide\",\"uuid\":\"6e43cbcf-e81f-4342-b8db-da903fa1233c\"},{\"content\":{\"side\":\"TOP\"},\"type\":\"ConnectorPlacement.EquallySpacedRectSide\",\"uuid\":\"1bde045f-2e19-44b2-bb97-f5d7a3b2c805\"},{\"content\":{\"connectorIds\":[\"RConn1\"],\"side\":\"BOTTOM\"},\"type\":\"ConnectorPlacement.EquallySpacedRectSide\",\"uuid\":\"cb3c2f40-1d14-4d09-ae00-a86e42d9c61f\"}]},\"type\":\"ConnectorPlacement.EquallySpacedConnector\",\"uuid\":\"58403efd-1890-4f51-bc4c-34e88e0faefd\"}],\"packageUris\":[\"http://schema.mathworks.com/mf0/Connector/R2020b\"],\"version\":\"1.0\"}"
  Right Hind Flipper : Subsystem
  SPS3 : nesl_utility/Simulink-PS Converter  PhysicalDomain=network_engine_domain  SubClassName=ps_input  LeftPortType=input  RightPortType=output  PseudoPeriodic=off  Frequencies=[]  NoiseDistribution=none  NoiseParameters=[]  Unit=N  AffineConversion=off  FilteringAndDerivatives=provide  SimscapeFilterOrder=1  InputFilterTimeConstant=0.001  UdotUserProvided=0
  Subsystem : Subsystem
  Tail Section Forces : Subsystem
  To Center : PMIOPort  Side=Left
  World Frame : PMIOPort  Port=2  Side=Left
  wires:
  Buoyancy (N)/1 -> SPS3/1
  connections:
  SPS3/RConn1 -- Fz on the CoB/LConn1
  Fz on the CoB/RConn1 -- Hind Flipper Connection/LConn4
  Tail Section Forces/LConn1 -- Left Hind Flipper/LConn1 -- World Frame/RConn1 -- Right Hind Flipper/RConn1
  Tail Section Forces/RConn1 -- Hind Flipper Connection/LConn3
  Hind Flipper Connection/RConn1 -- Left Hind Flipper/RConn1
  Right Hind Flipper/LConn1 -- Hind Flipper Connection/LConn2
  Hind Section Actuators/LConn1 -- To Center/RConn1
  Hind Flipper Connection/LConn1 -- Hind Section Actuators/RConn1
  Subsystem/LConn1 -- Hind Flipper Connection/RConn2

== system SEAMOUR_Sim/Sealion Robot/Subsystem ==
  Body Shell : sm_lib/Body Elements/File Solid  ExtGeomFileName=full_body_assem_06232023.stp  UnitType=FromFile  ExtGeomFileUnits=mm  StepReaderType=HEX  ExportConvexHullGeometry=off  InertiaType=Custom  Mass=center_body.mass  MassUnits=kg  CenterOfMass=center_body.com  CenterOfMassUnits=m  MomentsOfInertia=center_body.inertia  MomentsOfInertiaUnits=kg*m^2  ProductsOfInertia=center_body.prodinertia  ProductsOfInertiaUnits=kg*m^2  BasedOnType=Density  Density=1000  DensityUnits=kg/m^3  DoExposeReferenceFrame=off  SerializedFrames=<Frames><Frame><Id>Frame1</Id><Value><Name>Right</Name><Origin><Source>GeometricFeature</Source><FeatureName>circular curve 20</FeatureName></Origin><PrimaryAxis><DefinedDirection>-Z</DefinedDirection><Source>ReferenceFrame</Source><SourceDirection>+Y</SourceDirection><FeatureName></FeatureName></PrimaryAxis><SecondaryAxis><DefinedDirection>-Y</DefinedDirection><Source>ReferenceFrame</Source><SourceDirection>+X</SourceDirection><FeatureName></FeatureName></SecondaryAxis></Value></Frame><Frame><Id>Frame2</Id><Value><Name>Left</Name><Origin><Source>GeometricFeature</Source><FeatureName>circular curve 8</FeatureName></Origin><PrimaryAxis><DefinedDirection>+X</DefinedDirection><Source>ReferenceFrame</Source><SourceDirection>+Z</SourceDirection><FeatureName></FeatureName></PrimaryAxis><SecondaryAxis><DefinedDirection>-Y</DefinedDirection><Source>ReferenceFrame</Source><SourceDirection>+X</SourceDirection><FeatureName></FeatureName></SecondaryAxis></Value></Frame><Frame><Id>Frame3</Id><Value><Name>CoM</Name><Origin><Source>CenterOfMassFrame</Source><FeatureName></FeatureName></Origin><PrimaryAxis><DefinedDirection>+Z</DefinedDirection><Source>ReferenceFrame</Source><SourceDirection>+Z</SourceDirection><FeatureName></FeatureName></PrimaryAxis><SecondaryAxis><DefinedDirection>+X</DefinedDirection><Source>ReferenceFrame</Source><SourceDirection>+X</SourceDirection><FeatureName></FeatureName></SecondaryAxis></Value></Frame><Frame><Id>Frame4</Id><Value><Name>Head</Name><Origin><Source>GeometricFeature</Source><FeatureName>circular curve 16</FeatureName></Origin><PrimaryAxis><DefinedDirection>+Z</DefinedDirection><Source>ReferenceFrame</Source><SourceDirection>+Z</SourceDirection><FeatureName></FeatureName></PrimaryAxis><SecondaryAxis><DefinedDirection>+X</DefinedDirection><Source>ReferenceFrame</Source><SourceDirection>+X</SourceDirection><FeatureName></FeatureName></SecondaryAxis></Value></Frame><Frame><Id>Frame5</Id><Value><Name>Rear</Name><Origin><Source>GeometricFeature</Source><FeatureName>circular curve 178</FeatureName></Origin><PrimaryAxis><DefinedDirection>+X</DefinedDirection><Source>ReferenceFrame</Source><SourceDirection>+Z</SourceDirection><FeatureName></FeatureName></PrimaryAxis><SecondaryAxis><DefinedDirection>+Y</DefinedDirection><Source>ReferenceFrame</Source><SourceDirection>+X</SourceDirection><FeatureName></FeatureName></SecondaryAxis></Value></Frame><Frame><Id>Frame6</Id><Value><Name>Ref Frame</Name><Origin><Source>ReferenceFrame</Source><FeatureName></FeatureName></Origin><PrimaryAxis><DefinedDirection>+Z</DefinedDirection><Source>ReferenceFrame</Source><SourceDirection>+Z</SourceDirection><FeatureName></FeatureName></PrimaryAxis><SecondaryAxis><DefinedDirection>+X</DefinedDirection><Source>ReferenceFrame</Source><SourceDirection>+X</SourceDirection><FeatureName></FeatureName></SecondaryAxis></Value></Frame><Frame><Id>Frame7</Id><Value><Name>Geometric Center</Name><Origin><Source>GeometricFeature</Source><FeatureName>circular curve 101</FeatureName></Origin><PrimaryAxis><DefinedDirection>+Z</DefinedDirection><Source>ReferenceFrame</Source><SourceDirection>+Z</SourceDirection><FeatureName></FeatureName></PrimaryAxis><SecondaryAxis><DefinedDirection>+X</DefinedDirection><Source>ReferenceFrame</Source><SourceDirection>+X</SourceDirection><FeatureName></FeatureName></SecondaryAxis></Value></Frame></Frames>  GraphicType=FromGeometry  MarkerShape=Sphere  MarkerSize=10  GraphicVisPropType=SimpleVisualProperties  GraphicDiffuseColor=[0.2 0.4 1.0]  GraphicSpecularColor=[0.5 0.5 0.5 1.0]  GraphicAmbientColor=[0.15 0.15 0.15 1.0]  GraphicEmissiveColor=[0.0 0.0 0.0 1.0]  GraphicShininess=75  GraphicOpacity=0.25
  Ellipsoidal Solid : sm_lib/Body Elements/Ellipsoidal Solid  GraphicAmbientColor=[0.15 0.15 0.15 1.0]  BasedOnType=Density  CenterOfMass=[0 0 0]  CenterOfMassUnits=m  GraphicDiffuseColor=[0.5 0.5 0.5]  Density=0  DensityUnits=kg/m^3  DoExposeReferenceFrame=on  EllipsoidRadii=[.4 .115 .09]  EllipsoidRadiiUnits=m  GraphicEmissiveColor=[0.0 0.0 0.0 1.0]  ExportEntireGeometry=on  SerializedFrames=<Frames/>  MarkerShape=Sphere  MarkerSize=10  GraphicType=FromGeometry  InertiaType=CalculateFromGeometry  Mass=1  MassUnits=kg  MomentsOfInertia=[1 1 1]  MomentsOfInertiaUnits=kg*m^2  GraphicOpacity=0  ProductsOfInertia=[0 0 0]  ProductsOfInertiaUnits=kg*m^2  GraphicShininess=75  GraphicSpecularColor=[0.5 0.5 0.5 1.0]  GraphicVisPropType=SimpleVisualProperties
  To Right Flipper : PMIOPort  Side=Left
  To Head : PMIOPort  Port=2  Side=Left
  To Left Flipper : PMIOPort  Port=3  Side=Right
  CoM : PMIOPort  Port=4  Side=Right
  To Rear : PMIOPort  Port=5  Side=Right
  To Ref : PMIOPort  Port=6  Side=Right
  Center Hull Boundary : PMIOPort  Port=7  Side=Right
  connections:
  Body Shell/LConn1 -- To Right Flipper/RConn1
  Body Shell/LConn3 -- To Rear/RConn1
  Body Shell/LConn2 -- CoM/RConn1
  Body Shell/RConn1 -- To Left Flipper/RConn1
  Body Shell/RConn2 -- To Head/RConn1
  To Ref/RConn1 -- Body Shell/RConn3
  Ellipsoidal Solid/RConn1 -- Body Shell/LConn4
  Center Hull Boundary/RConn1 -- Ellipsoidal Solid/LConn1
